simulink model "sensor_model"  (R2018a)
settings: Solver=FixedStepAuto  StartTime=0.0  StopTime=400  RelTol=1e-3
libraries: simulink x2
settings Model: Creator=cory0  LastModifiedBy=xzhang

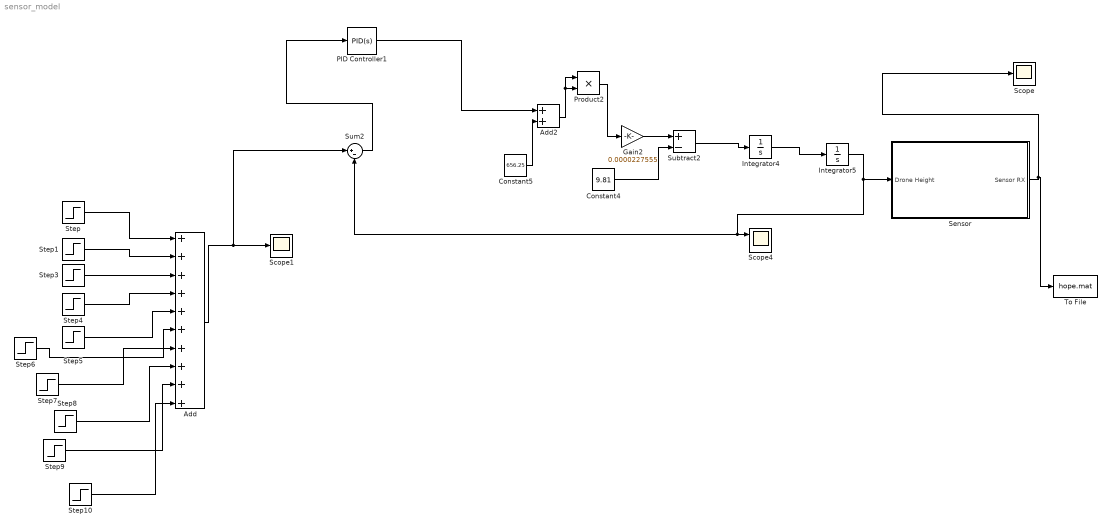
== system sensor_model ==
  Add : Sum  Inputs=++++++++++
  Add2 : Sum
  Constant4 : Constant  Value=9.81
  Constant5 : Constant  Value=656.25
  Gain2 : Gain  Gain=0.0000227555
  Integrator4 : Integrator
  Integrator5 : Integrator
  PID Controller1 : simulink/Continuous/PID Controller  Controller=PID  TimeDomain=Continuous-time  SampleTime=-1  IntegratorMethod=Forward Euler  FilterMethod=Forward Euler  Form=Parallel  UseFilter=on  ControllerParametersSource=internal  P=80  I=2  D=84  N=10  InitialConditionSource=internal  InitialConditionForIntegrator=0  InitialConditionForFilter=0  ExternalReset=none  LimitOutput=off  UpperSaturationLimit=inf  LowerSaturationLimit=-inf  LinearizeAsGain=on  AntiWindupMode=none  Kb=1  TrackingMode=off  Kt=1  PParamMin=[]  PParamMax=[]  IParamMin=[]  IParamMax=[]  DParamMin=[]  DParamMax=[]  NParamMin=[]  NParamMax=[]  KbParamMin=[]  KbParamMax=[]  KtParamMin=[]  KtParamMax=[]  POutMin=[]  POutMax=[]  IOutMin=[]  IOutMax=[]  DOutMin=[]  DOutMax=[]  NOutMin=[]  NOutMax=[]  KbOutMin=[]  KbOutMax=[]  KtOutMin=[]  KtOutMax=[]  IntegratorOutMin=[]  IntegratorOutMax=[]  FilterOutMin=[]  FilterOutMax=[]  SumOutMin=[]  SumOutMax=[]  SumI1OutMin=[]  SumI1OutMax=[]  SumI2OutMin=[]  SumI2OutMax=[]  SumI3OutMin=[]  SumI3OutMax=[]  SumDOutMin=[]  SumDOutMax=[]  SaturationOutMin=[]  SaturationOutMax=[]  IntegratorContinuousStateAttributes=''  IntegratorStateMustResolveToSignalObject=off  IntegratorRTWStateStorageClass=Auto  FilterContinuousStateAttributes=''  FilterStateMustResolveToSignalObject=off  FilterRTWStateStorageClass=Auto  DifferentiatorICPrevScaledInput=0  DifferentiatorOutMin=[]  DifferentiatorOutMax=[]  FilterDiffOutCoefMin=[]  FilterDiffOutCoefMax=[]  SumDenOutMin=[]  SumDenOutMax=[]  SumNumOutMin=[]  SumNumOutMax=[]  ReciprocalOutMin=[]  ReciprocalOutMax=[]  DivideOutMin=[]  DivideOutMax=[]  TunerSelectOption=Transfer Function Based (PID Tuner App)
  Product2 : Product
  Scope : Scope
  Scope1 : Scope
  Scope4 : Scope  NumInputPorts=2
  Sensor : Subsystem
  Step : Step  Time=0  SampleTime=0
  Step1 : Step  Time=40  SampleTime=0
  Step10 : Step  Time=360  SampleTime=0
  Step3 : Step  Time=80  SampleTime=0
  Step4 : Step  Time=120  SampleTime=0
  Step5 : Step  Time=160  SampleTime=0
  Step6 : Step  Time=200  SampleTime=0
  Step7 : Step  Time=240  SampleTime=0
  Step8 : Step  Time=280  SampleTime=0
  Step9 : Step  Time=320  SampleTime=0
  Subtract2 : Sum  Inputs=+-
  Sum2 : Sum  Inputs=|+-
  To File : ToFile  Filename=hope.mat
  wires:
  PID Controller1/1 -> Add2/1
  Sum2/1 -> PID Controller1/1
  Integrator4/1 -> Integrator5/1
  Gain2/1 -> Subtract2/1
  Constant5/1 -> Add2/2
  Product2/1 -> Gain2/1
  Add2/1 -> Product2/2, Product2/1
  Subtract2/1 -> Integrator4/1
  Integrator5/1 -> Sensor/1(Drone Height), Scope4/1, Sum2/2
  Constant4/1 -> Subtract2/2
  Sensor/1(Sensor RX) -> To File/1, Scope/1
  Add/1 -> Sum2/1, Scope1/1
  Step1/1 -> Add/2
  Step/1 -> Add/1
  Step3/1 -> Add/3
  Step4/1 -> Add/4
  Step5/1 -> Add/5
  Step6/1 -> Add/6
  Step7/1 -> Add/7
  Step8/1 -> Add/8
  Step9/1 -> Add/9
  Step10/1 -> Add/10

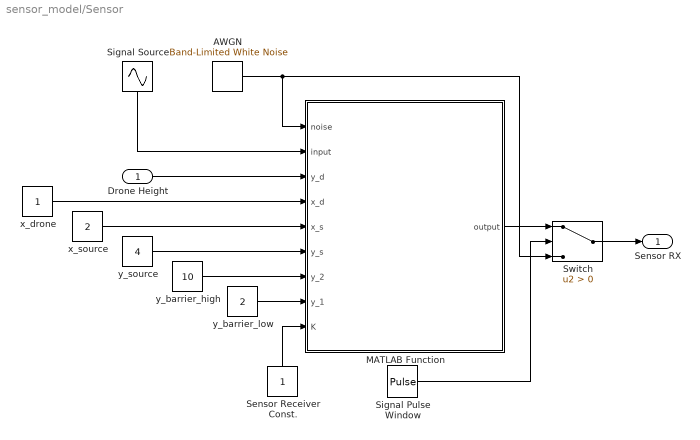
== system sensor_model/Sensor ==
  Drone Height : Inport
  AWGN : simulink/Sources/Band-Limited White Noise  Cov=[0.00001]  Ts=0.0005  seed=[23340]
  MATLAB Function : MATLAB Function  TreatAsAtomicUnit=on
  Sensor Receiver Const. : Constant
  Signal Source : Sin  Amplitude=10  Frequency=6.2831853  SampleTime=0
  Signal Pulse Window : DiscretePulseGenerator  PulseType=Time based  Period=20  PulseWidth=75
  Switch : Switch  Criteria=u2 > Threshold
  x_drone : Constant
  x_source : Constant  Value=2
  y_barrier_high : Constant  Value=10
  y_barrier_low : Constant  Value=2
  y_source : Constant  Value=4
  Sensor RX : Outport
  wires:
  Sensor Receiver Const./1 -> MATLAB Function/9(K)
  Signal Source/1 -> MATLAB Function/2(input)
  Signal Pulse Window/1 -> Switch/2
  y_source/1 -> MATLAB Function/6(y_s)
  y_barrier_low/1 -> MATLAB Function/8(y_1)
  x_drone/1 -> MATLAB Function/4(x_d)
  MATLAB Function/1(output) -> Switch/1
  AWGN/1 -> MATLAB Function/1(noise), Switch/3
  y_barrier_high/1 -> MATLAB Function/7(y_2)
  x_source/1 -> MATLAB Function/5(x_s)
  Drone Height/1 -> MATLAB Function/3(y_d)
  Switch/1 -> Sensor RX/1

== matlab function sensor_model/Sensor/MATLAB Function ==
  data: noise input; input input; y_d input; x_d input; output output; x_s input; y_s input; y_2 input; y_1 input; K input
function output = sensor_filter(noise,input,y_d,x_d,x_s,y_s,y_2,y_1,K)
    
    % Line of Sight Aperture
    c = y_d + (y_s-y_d)*x_d/(x_s+x_d);
    
    % Drone-Sensor Distance
    d = sqrt((x_d+x_s)^2 + (y_d-y_s)^2);
    
    % Sensor Reading
    if (c >= y_1) && (c <= y_2)
        output = sqrt(K)*input/d + noise;
    else
        output = noise;
    end

end
